simulink model "SLDTAREA"  (R2023a)
settings: Solver=VariableStepAuto  StartTime=0.0  StopTime=60  MaxStep=0.01  RelTol=1e-3
values from neighbouring files (symbols this model uses):
  c1 = f2-f1    (= 1000)    [SLDTAREACODE.m]
  c2 = (2*pi*f_0)/(c1)    (= 0.00314159265359)    [SLDTAREACODE.m]
  da = 2000    [SLDTAREACODE.m]
  f1 = 5000    [SLDTAREACODE.m]
  f2 = 6000    [SLDTAREACODE.m]
  f3 = 4000    [SLDTAREACODE.m]
  kr = 20000    [SLDTAREACODE.m]
  m = 5000    [SLDTAREACODE.m]
  p = (f2-f3)/10    (= 200)    [SLDTAREACODE.m]
libraries: simulink x13
settings Model: NumberOfSteps=10  Creator=mluser  LastModifiedBy=fabia

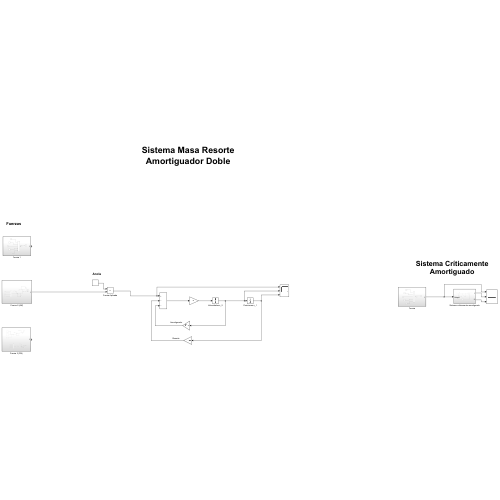
[thumbnail: Simulink's stored preview of the top-level diagram]
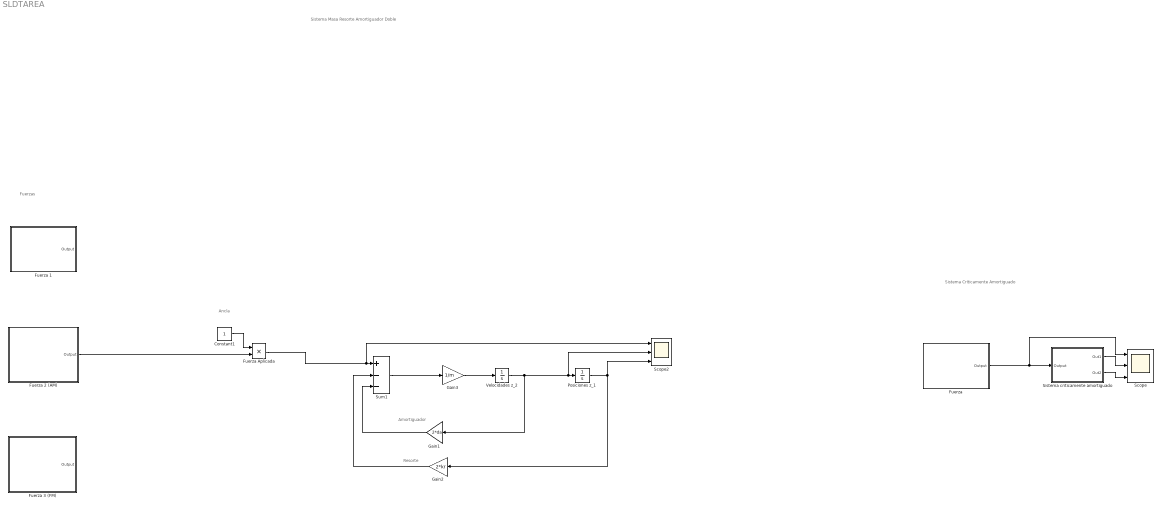
== system SLDTAREA ==
  note: Sistema Masa Resorte Amortiguador Doble
  note: Fuerzas
  note: Sistema Críticamente Amortiguado
  note: Resorte
  note: Amortiguador
  note: Ancla
  Constant1 : Constant
  Fuerza : Subsystem
  Fuerza 1 : Subsystem
  Fuerza 2 (AM) : Subsystem
  Fuerza 3 (FM) : Subsystem
  Fuerza Aplicada : Product
  Gain1 : Gain  Gain=2*da
  Gain2 : Gain  Gain=2*kr
  Gain3 : Gain  Gain=1/m
  Posiciones z_1 : Integrator
  Scope : Scope  NumInputPorts=3
  Scope2 : Scope  NumInputPorts=3
  Sistema criticamente amortiguado : Subsystem
  Sum1 : Sum  Inputs=+--
  Velocidades z_2 : Integrator
  wires:
  Fuerza/1(Output) -> Scope/1, Sistema criticamente amortiguado/1(Output)
  Sistema criticamente amortiguado/1(Out1) -> Scope/2
  Sistema criticamente amortiguado/2(Out2) -> Scope/3
  Fuerza Aplicada/1 -> Scope2/1, Sum1/1
  Constant1/1 -> Fuerza Aplicada/1
  Gain1/1 -> Sum1/3
  Gain3/1 -> Velocidades z_2/1
  Gain2/1 -> Sum1/2
  Sum1/1 -> Gain3/1
  Velocidades z_2/1 -> Scope2/2, Posiciones z_1/1, Gain1/1
  Fuerza 2 (AM)/1(Output) -> Fuerza Aplicada/2
  Posiciones z_1/1 -> Gain2/1, Scope2/3

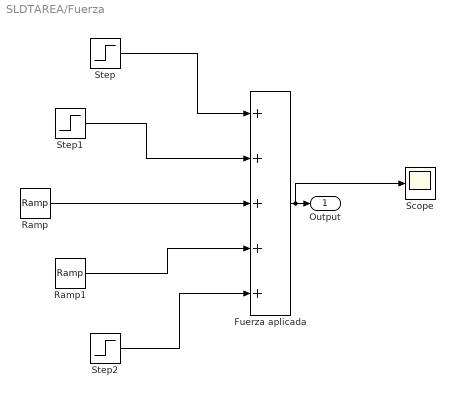
== system SLDTAREA/Fuerza ==
  Fuerza aplicada : Sum  Inputs=+++++
  Ramp : simulink/Sources/Ramp  slope=-p  start=20  InitialOutput=0
  Ramp1 : simulink/Sources/Ramp  slope=p  start=30  InitialOutput=0
  Scope : Scope
  Step : Step  Time=0  After=f1  SampleTime=0
  Step1 : Step  Time=5  After=(f2-f1)  SampleTime=0
  Step2 : Step  Time=45  After=f1-f3  SampleTime=0
  Output : Outport
  wires:
  Step2/1 -> Fuerza aplicada/5
  Ramp1/1 -> Fuerza aplicada/4
  Step1/1 -> Fuerza aplicada/2
  Ramp/1 -> Fuerza aplicada/3
  Step/1 -> Fuerza aplicada/1
  Fuerza aplicada/1 -> Scope/1, Output/1

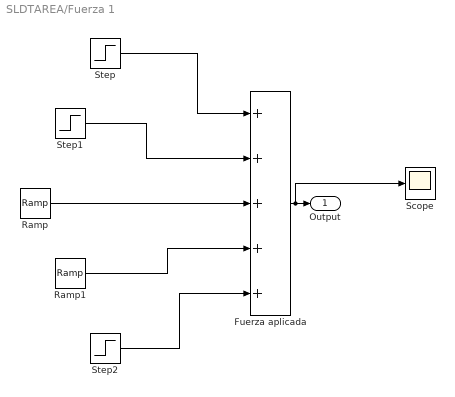
== system SLDTAREA/Fuerza 1 ==
  Fuerza aplicada : Sum  Inputs=+++++
  Ramp : simulink/Sources/Ramp  slope=-p  start=20  InitialOutput=0
  Ramp1 : simulink/Sources/Ramp  slope=p  start=30  InitialOutput=0
  Scope : Scope
  Step : Step  Time=0  After=f1  SampleTime=0
  Step1 : Step  Time=5  After=(f2-f1)  SampleTime=0
  Step2 : Step  Time=45  After=f1-f3  SampleTime=0
  Output : Outport
  wires:
  Step2/1 -> Fuerza aplicada/5
  Ramp1/1 -> Fuerza aplicada/4
  Step1/1 -> Fuerza aplicada/2
  Ramp/1 -> Fuerza aplicada/3
  Step/1 -> Fuerza aplicada/1
  Fuerza aplicada/1 -> Scope/1, Output/1

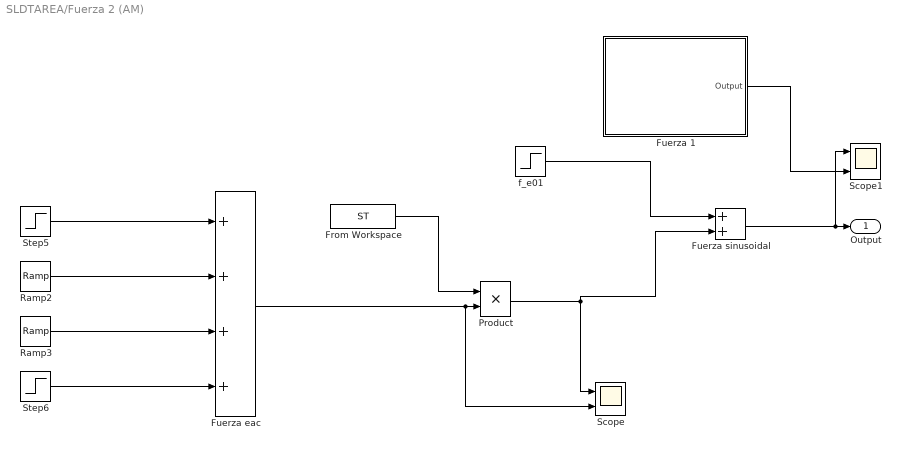
== system SLDTAREA/Fuerza 2 (AM) ==
  From Workspace : FromWorkspace  VariableName=ST
  Fuerza 1 : Subsystem
  Fuerza eac : Sum  Inputs=++++
  Fuerza sinusoidal : Sum
  Product : Product
  Ramp2 : simulink/Sources/Ramp  slope=-p  start=20  InitialOutput=0
  Ramp3 : simulink/Sources/Ramp  slope=p  start=30  InitialOutput=0
  Scope : Scope  NumInputPorts=2
  Scope1 : Scope  NumInputPorts=2
  Step5 : Step  Time=5  After=f2-f1  SampleTime=0
  Step6 : Step  Time=45  After=f1-f3  SampleTime=0
  f_e01 : Step  Time=0  After=f1  SampleTime=0
  Output : Outport
  wires:
  f_e01/1 -> Fuerza sinusoidal/1
  Fuerza eac/1 -> Scope/2, Product/2
  Product/1 -> Scope/1, Fuerza sinusoidal/2
  Step5/1 -> Fuerza eac/1
  Ramp2/1 -> Fuerza eac/2
  Step6/1 -> Fuerza eac/4
  Ramp3/1 -> Fuerza eac/3
  Fuerza sinusoidal/1 -> Scope1/1, Output/1
  From Workspace/1 -> Product/1
  Fuerza 1/1(Output) -> Scope1/2

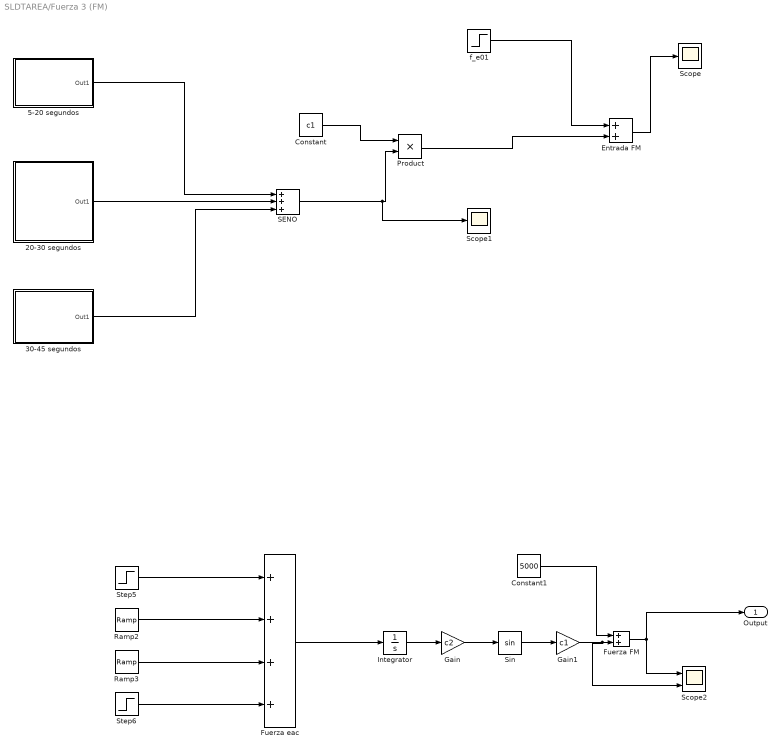
== system SLDTAREA/Fuerza 3 (FM) ==
  20-30 segundos : Subsystem
  30-45 segundos : Subsystem
  5-20 segundos : Subsystem
  Constant : Constant  Value=c1
  Constant1 : Constant  Value=5000
  Entrada FM : Sum
  Fuerza FM : Sum
  Fuerza eac : Sum  Inputs=++++
  Gain : Gain  Gain=c2
  Gain1 : Gain  Gain=c1
  Integrator : Integrator
  Product : Product
  Ramp2 : simulink/Sources/Ramp  slope=-p  start=20  InitialOutput=0
  Ramp3 : simulink/Sources/Ramp  slope=p  start=30  InitialOutput=0
  SENO : Sum  Inputs=+++
  Scope : Scope
  Scope1 : Scope
  Scope2 : Scope  NumInputPorts=2
  Sin : Trigonometry
  Step5 : Step  Time=5  After=f2-f1  SampleTime=0
  Step6 : Step  Time=45  After=f1-f3  SampleTime=0
  f_e01 : Step  Time=0  After=f1  SampleTime=0
  Output : Outport
  wires:
  f_e01/1 -> Entrada FM/1
  Entrada FM/1 -> Scope/1
  5-20 segundos/1(Out1) -> SENO/1
  20-30 segundos/1(Out1) -> SENO/2
  30-45 segundos/1(Out1) -> SENO/3
  SENO/1 -> Scope1/1, Product/2
  Constant/1 -> Product/1
  Product/1 -> Entrada FM/2
  Step5/1 -> Fuerza eac/1
  Ramp2/1 -> Fuerza eac/2
  Step6/1 -> Fuerza eac/4
  Ramp3/1 -> Fuerza eac/3
  Fuerza eac/1 -> Integrator/1
  Integrator/1 -> Gain/1
  Gain/1 -> Sin/1
  Sin/1 -> Gain1/1
  Gain1/1 -> Scope2/2, Fuerza FM/2
  Constant1/1 -> Fuerza FM/1
  Fuerza FM/1 -> Output/1, Scope2/1

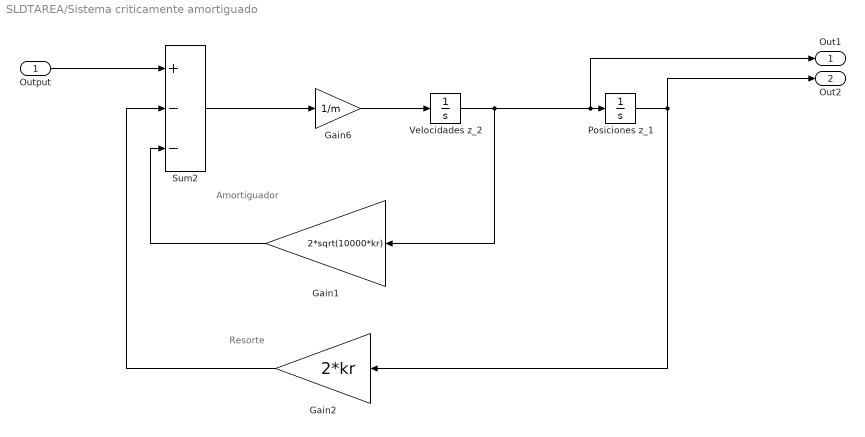
== system SLDTAREA/Sistema criticamente amortiguado ==
  note: Amortiguador
  note: Resorte
  Output : Inport
  Gain1 : Gain  Gain=2*sqrt(10000*kr)
  Gain2 : Gain  Gain=2*kr
  Gain6 : Gain  Gain=1/m
  Posiciones z_1 : Integrator
  Sum2 : Sum  Inputs=+--
  Velocidades z_2 : Integrator
  Out1 : Outport
  Out2 : Outport  Port=2
  wires:
  Gain2/1 -> Sum2/2
  Gain1/1 -> Sum2/3
  Velocidades z_2/1 -> Out1/1, Posiciones z_1/1, Gain1/1
  Posiciones z_1/1 -> Out2/1, Gain2/1
  Gain6/1 -> Velocidades z_2/1
  Sum2/1 -> Gain6/1
  Output/1 -> Sum2/1

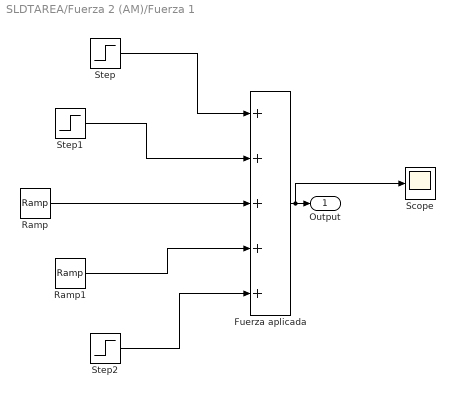
== system SLDTAREA/Fuerza 2 (AM)/Fuerza 1 ==
  Fuerza aplicada : Sum  Inputs=+++++
  Ramp : simulink/Sources/Ramp  slope=-p  start=20  InitialOutput=0
  Ramp1 : simulink/Sources/Ramp  slope=p  start=30  InitialOutput=0
  Scope : Scope
  Step : Step  Time=0  After=f1  SampleTime=0
  Step1 : Step  Time=5  After=(f2-f1)  SampleTime=0
  Step2 : Step  Time=45  After=f1-f3  SampleTime=0
  Output : Outport
  wires:
  Step2/1 -> Fuerza aplicada/5
  Ramp1/1 -> Fuerza aplicada/4
  Step1/1 -> Fuerza aplicada/2
  Ramp/1 -> Fuerza aplicada/3
  Step/1 -> Fuerza aplicada/1
  Fuerza aplicada/1 -> Scope/1, Output/1

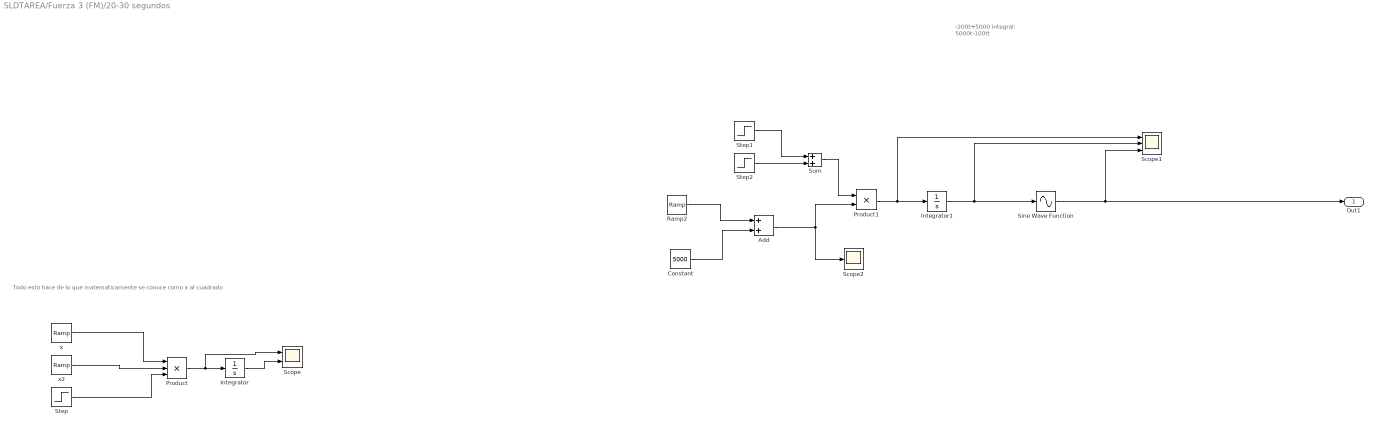
== system SLDTAREA/Fuerza 3 (FM)/20-30 segundos ==
  note: -200t+5000
      | integral:
      | 5000t-100tt
  note: Todo esto hace de lo que matematicamente se conoce como x al cuadrado
  Add : Sum
  Constant : Constant  Value=5000
  Integrator : Integrator  LimitOutput=on  LowerSaturationLimit=0
  Integrator1 : Integrator
  Product : Product  Inputs=3
  Product1 : Product
  Ramp2 : simulink/Sources/Ramp  slope=-200  start=0  InitialOutput=0
  Scope : Scope  NumInputPorts=2
  Scope1 : Scope  NumInputPorts=3
  Scope2 : Scope
  Sine Wave Function : Sin  TimeSource=Use external signal  SampleTime=0
  Step : Step  Time=0  SampleTime=0
  Step1 : Step  Time=20  SampleTime=0
  Step2 : Step  Time=30  After=-1  SampleTime=0
  Sum : Sum
  x : simulink/Sources/Ramp  slope=1  start=0  InitialOutput=0
  x2 : simulink/Sources/Ramp  slope=1  start=0  InitialOutput=0
  Out1 : Outport
  wires:
  Integrator/1 -> Scope/2
  Step/1 -> Product/3
  x/1 -> Product/1
  Product/1 -> Integrator/1, Scope/1
  x2/1 -> Product/2
  Ramp2/1 -> Add/1
  Constant/1 -> Add/2
  Step2/1 -> Sum/2
  Step1/1 -> Sum/1
  Product1/1 -> Integrator1/1, Scope1/1
  Sum/1 -> Product1/1
  Add/1 -> Scope2/1, Product1/2
  Integrator1/1 -> Sine Wave Function/1, Scope1/2
  Sine Wave Function/1 -> Out1/1, Scope1/3

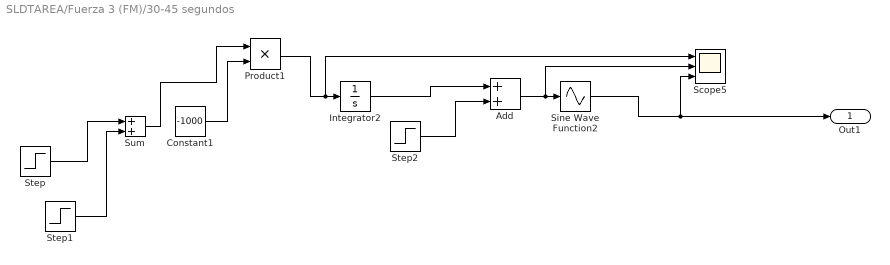
== system SLDTAREA/Fuerza 3 (FM)/30-45 segundos ==
  Add : Sum
  Constant1 : Constant  Value=-1000
  Integrator2 : Integrator
  Product1 : Product
  Scope5 : Scope  NumInputPorts=3
  Sine Wave Function2 : Sin  TimeSource=Use external signal  SampleTime=0
  Step : Step  Time=30  SampleTime=0
  Step1 : Step  Time=45  After=-1  SampleTime=0
  Step2 : Step  Time=45  After=-15000  SampleTime=0
  Sum : Sum
  Out1 : Outport
  wires:
  Step/1 -> Sum/1
  Step1/1 -> Sum/2
  Sum/1 -> Product1/1
  Constant1/1 -> Product1/2
  Integrator2/1 -> Add/1
  Add/1 -> Scope5/2, Sine Wave Function2/1
  Product1/1 -> Scope5/1, Integrator2/1
  Step2/1 -> Add/2
  Sine Wave Function2/1 -> Out1/1, Scope5/3

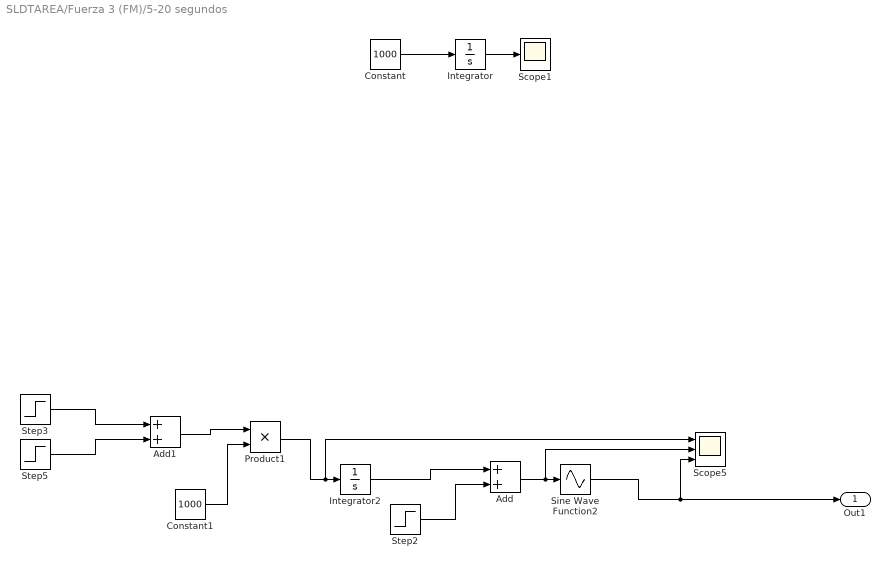
== system SLDTAREA/Fuerza 3 (FM)/5-20 segundos ==
  Add : Sum
  Add1 : Sum
  Constant : Constant  Value=1000
  Constant1 : Constant  Value=1000
  Integrator : Integrator  InitialCondition=5  LimitOutput=on  UpperSaturationLimit=10  LowerSaturationLimit=5
  Integrator2 : Integrator
  Product1 : Product
  Scope1 : Scope
  Scope5 : Scope  NumInputPorts=3
  Sine Wave Function2 : Sin  TimeSource=Use external signal  SampleTime=0
  Step2 : Step  Time=20  After=-15000  SampleTime=0
  Step3 : Step  Time=5  SampleTime=0
  Step5 : Step  Time=20  After=-1  SampleTime=0
  Out1 : Outport
  wires:
  Constant/1 -> Integrator/1
  Integrator/1 -> Scope1/1
  Step3/1 -> Add1/1
  Step5/1 -> Add1/2
  Sine Wave Function2/1 -> Scope5/3, Out1/1
  Product1/1 -> Scope5/1, Integrator2/1
  Add1/1 -> Product1/1
  Constant1/1 -> Product1/2
  Add/1 -> Scope5/2, Sine Wave Function2/1
  Integrator2/1 -> Add/1
  Step2/1 -> Add/2
